simulink library "M160_lib"  (Simulink 7.8)
settings: Solver=FixedStepDiscrete  StartTime=0.0  StopTime=10.0  RelTol=1e-3
PreLoadFcn:
  | update_path
undefined symbols (not defined in the file): Afr_atCool2facLambdaReqCorr_CUR_x, Afr_atCool2facLambdaReqCorr_CUR_y, Afr_atMani2facLambdaReqCorr_CUR_x, Afr_atMani2facLambdaReqCorr_CUR_y, Afr_facLambdaReqMan, Afr_facRatioMan, Afr_facStoich, Afr_flgLambdaReqOverride, Afr_flgRatioOverride, Afr_rpmEngSpdfacRelAir2facLambdaReqBase_MAP_x, Afr_rpmEngSpdfacRelAir2facLambdaReqBase_MAP_y, Afr_rpmEngSpdfacRelAir2facLambdaReqBase_MAP_z, Ais_flgAirInjReacPumpOverride, Ais_stAirInjReacPumpMan, Amc_flgAirMassFlowOverride, Amc_uSens2AirMassFlow_CUR_x, Amc_uSens2AirMassFlow_CUR_y, Amc_uSensMaxValid, Amc_uSensMinValid, Amf_facRelAirMan, Amf_flgAirMassPerStrOverride, Amf_flgRelAirOverride, Amf_flgSwitch2AirMassFlowMeter, Amf_mAirPerStrMan, Amf_pManiEngSpd2facRelAirCorr_MAP_x, Amf_pManiEngSpd2facRelAirCorr_MAP_y, Amf_pManiEngSpd2facRelAirCorr_MAP_z, Amf_rpmEngSpd2facTempCorr_CUR_x, Amf_rpmEngSpd2facTempCorr_CUR_y, Amf_shcSpecGasConst_C, Amf_volEngDisp_C, Apv_facAirPumpRateMan, Apv_factor, Apv_flgAirPumpRateOverride, Apv_tiPeriod_C, Bvc_rVoltDivHigh, Bvc_rVoltDivLow, Bvc_uBattMax, Bvc_uBattMin, CDRV_E_OK_, Cov_facChOverVlvRateMan, Cov_factor, Cov_flgChOverVlvRateOverride, Cov_tiPeriod_C, Cpc_atManiTmp2facPresCorr_CUR_x, Cpc_atManiTmp2facPresCorr_CUR_y, Cpc_flgPChargeOverride, Cpc_uSens2pManiBase_CUR_x, Cpc_uSens2pManiBase_CUR_y, Ctc_rPullUp_C, Ctc_rSens2atCool_CUR_x, Ctc_rSens2atCool_CUR_y, Ctc_uSensMaxValid, Ctc_uSensMinValid, Ctc_uSupply, Doh_OutputDiagnosisOverride, dummy_facAirPumpRateReq, dummy_facChOverVlvRateReq, dummy_flgInterCoolerOverride, dummy_flgKl50Override ... (+243)
libraries: simulink x36, ehooks_lib x3
(part 3 of 8)

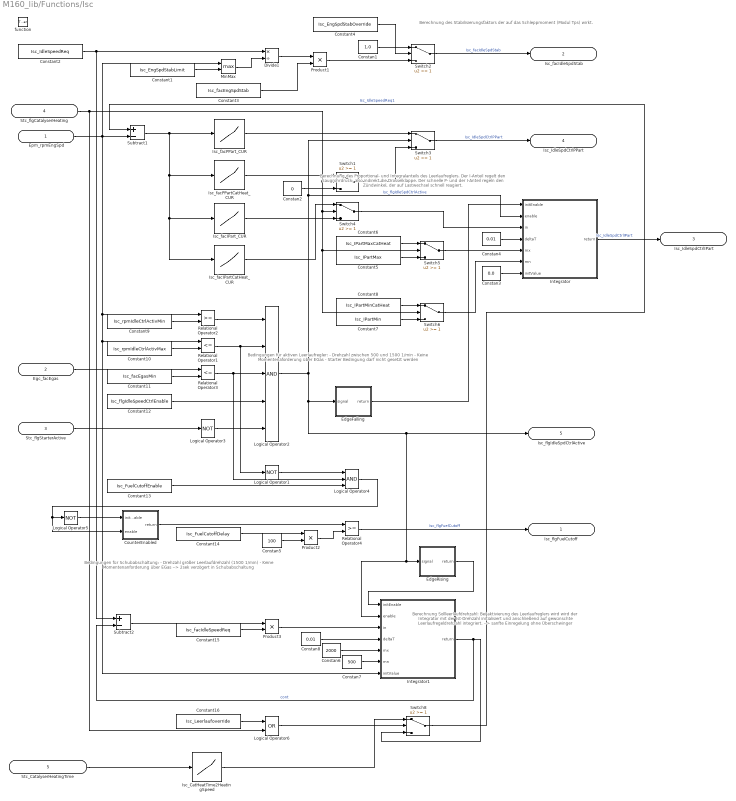
== system M160_lib/Functions/Isc ==
  note: Berechnung des Stabilisierungsfaktors der auf das Schleppmoment (Modul Tps) wirkt.
  note: Berechnung des Proportional- und Integralanteils des Leerlaufreglers.
      | Der I-Anteil regelt den Saugrohrdruck, also indirekt die Drosselklappe.
      | Der schnelle P- und der I-Anteil regeln den Zündwinkel, der auf
      | Lastwechsel schnell reagiert.
  note: Bedingungen für aktiven Leerlaufregler:
      | - Drehzahl zwischen 500 und 1500 1/min
      | - Keine Momentenaforderung über EGas
      | - Starter Bedingung darf nicht gesetzt werden
  note: Bedingungen für Schubabschaltung:
      | - Drehzahl größer Leerlaufdrehzahl (1500 1/min)
      | - Keine Momentenanforderung über EGas
      | --> 2sek verzögert in Schubabschaltung
  note: Berechnung Sollleerlaufdrehzahl:
      | Bei aktivierung des Leerlaufreglers wird
      | wird der Integrator mit der Ist-Drehzahl
      | initialisiert und anschließend auf gewünschte
      | Leerlaufregeldrehzahl integriert.
      | --> sanfte Einregelung ohne Überschwinger
  Epm_rpmEngSpd : Inport
  Egc_facEgas : Inport  Port=2
  Stc_flgStarterActive : Inport  Port=3
  Stc_flgCatalyserHeating : Inport  Port=4
  Stc_CatalyserHeatingTime : Inport  Port=5
  function : TriggerPort  TriggerType=function-call
  Constan1 : Constant  Value=1.0  OutDataTypeStr=single
  Constan2 : Constant  Value=0  OutDataTypeStr=single
  Constan3 : Constant  Value=0.0  OutDataTypeStr=single
  Constan4 : Constant  Value=0.01  OutDataTypeStr=single
  Constan5 : Constant  Value=100  OutDataTypeStr=single
  Constan6 : Constant  Value=2000  OutDataTypeStr=single
  Constan7 : Constant  Value=500  OutDataTypeStr=single
  Constan8 : Constant  Value=0.01  OutDataTypeStr=single
  Constant1 : Constant  Value=Isc_EngSpdStabLimit
  Constant10 : Constant  Value=Isc_rpmIdleCtrlActivMax
  Constant11 : Constant  Value=Isc_facEgasMin
  Constant12 : Constant  Value=Isc_flgIdleSpeedCtrlEnable
  Constant13 : Constant  Value=Isc_FuelCutoffEnable
  Constant14 : Constant  Value=Isc_FuelCutoffDelay
  Constant15 : Constant  Value=Isc_facIdleSpeedReq
  Constant16 : Constant  Value=Isc_Leerlaufoverride
  Constant2 : Constant  Value=Isc_IdleSpeedReq
  Constant3 : Constant  Value=Isc_facEngSpdStab
  Constant4 : Constant  Value=Isc_EngSpdStabOverride
  Constant5 : Constant  Value=Isc_IPartMax
  Constant6 : Constant  Value=Isc_IPartMaxCatHeat
  Constant7 : Constant  Value=Isc_IPartMin
  Constant8 : Constant  Value=Isc_IPartMinCatHeat
  Constant9 : Constant  Value=Isc_rpmIdleCtrlActivMin
  CounterEnabled : Subsystem
      mask Description: Counter
      mask Display: image(imread('CounterEnabled.jpg'))
  Divide1 : Product  Inputs=*/  OutDataTypeStr=Inherit: Same as first input
  EdgeFalling : Subsystem
      mask Description: EdgeFalling
      mask Display: image(imread('EdgeFalling.jpg'))
  EdgeRising : Subsystem
      mask Description: EdgeRising
      mask Display: image(imread('EdgeRising.jpg'))
  Integrator : Subsystem
      mask Description: Integrator
      mask Display: image(imread('Integrator.jpg'))
  Integrator1 : Subsystem
      mask Description: Integrator
      mask Display: image(imread('Integrator.jpg'))
  Isc_CatHeatTime2HeatingSpeed : Lookup_n-D  NumberOfTableDimensions=1  BreakpointsForDimension1=Isc_CatHeatTime2HeatingSpeed_x  Table=Isc_CatHeatTime2HeatingSpeed_y  ExtrapMethod=Clip  InputSameDT=on
  Isc_facIPartCatHeat_CUR : Lookup_n-D  NumberOfTableDimensions=1  BreakpointsForDimension1=Isc_facIPartCatHeat_CUR_x  Table=Isc_facIPartCatHeat_CUR_y  ExtrapMethod=Clip  InputSameDT=on
  Isc_facIPart_CUR : Lookup_n-D  NumberOfTableDimensions=1  BreakpointsForDimension1=Isc_facIPart_CUR_x  Table=Isc_facIPart_CUR_y  ExtrapMethod=Clip  InputSameDT=on
  Isc_facPPartCatHeat_CUR : Lookup_n-D  NumberOfTableDimensions=1  BreakpointsForDimension1=Isc_facPPartCatHeat_CUR_x  Table=Isc_facPPartCatHeat_CUR_y  ExtrapMethod=Clip  InputSameDT=on
  Isc_facPPart_CUR : Lookup_n-D  NumberOfTableDimensions=1  BreakpointsForDimension1=Isc_facPPart_CUR_x  Table=Isc_facPPart_CUR_y  ExtrapMethod=Clip  InputSameDT=on
  Logical Operator1 : Logic  Operator=NOT  AllPortsSameDT=off  OutDataTypeStr=boolean
  Logical Operator2 : Logic  Inputs=5  AllPortsSameDT=off  OutDataTypeStr=boolean
  Logical Operator3 : Logic  Operator=NOT  AllPortsSameDT=off  OutDataTypeStr=boolean
  Logical Operator4 : Logic  Inputs=3  AllPortsSameDT=off  OutDataTypeStr=boolean
  Logical Operator5 : Logic  Operator=NOT  AllPortsSameDT=off  OutDataTypeStr=boolean
  Logical Operator6 : Logic  Operator=OR  AllPortsSameDT=off  OutDataTypeStr=boolean
  MinMax : MinMax  Function=max  Inputs=2
  Product1 : Product  OutDataTypeStr=Inherit: Same as first input
  Product2 : Product  OutDataTypeStr=Inherit: Same as first input
  Product3 : Product  OutDataTypeStr=Inherit: Same as first input
  Relational Operator1 : RelationalOperator  Operator=<=  OutDataTypeStr=boolean
  Relational Operator2 : RelationalOperator  OutDataTypeStr=boolean
  Relational Operator3 : RelationalOperator  Operator=<=  OutDataTypeStr=boolean
  Relational Operator4 : RelationalOperator  OutDataTypeStr=boolean
  Subtract1 : Sum  Inputs=+-  OutDataTypeStr=Inherit: Same as first input
  Subtract2 : Sum  Inputs=+-  OutDataTypeStr=Inherit: Same as first input
  Switch{1..6,8} (7 alike) : Switch  Threshold=1
  Isc_flgFuelCutoff : Outport
  Isc_facIdleSpdStab : Outport  Port=2
  Isc_IdleSpdCtrlIPart : Outport  Port=3
  Isc_IdleSpdCtrlPPart : Outport  Port=4
  Isc_flgIdleSpdCtrlActive : Outport  Port=5
  wires:
  Constant2/1 -> Divide1/1, Subtract2/1
  MinMax/1 -> Divide1/2
  Constant1/1 -> MinMax/2
  Epm_rpmEngSpd/1 -> MinMax/1, Subtract1/2, Relational Operator2/1, Relational Operator1/1, Integrator1/7(initValue)
  Divide1/1 -> Product1/1
  Constant3/1 -> Product1/2
  Product1/1 -> Switch2/3
  Constan1/1 -> Switch2/1
  Constant4/1 -> Switch2/2
  Switch2/1 -> Isc_facIdleSpdStab/1  "Isc_facIdleSpdStab"
  Subtract1/1 -> Isc_facPPart_CUR/1, Isc_facPPartCatHeat_CUR/1, Isc_facIPart_CUR/1, Isc_facIPartCatHeat_CUR/1
  Constan2/1 -> Switch1/3
  Switch1/1 -> Switch3/3
  Switch3/1 -> Isc_IdleSpdCtrlPPart/1  "Isc_IdleSpdCtrlPPart"
  Stc_flgCatalyserHeating/1 -> Switch1/2, Switch4/2, Switch5/2, Switch6/2, Logical Operator6/2
  Isc_facPPartCatHeat_CUR/1 -> Switch1/1
  Isc_facPPart_CUR/1 -> Switch3/1
  Integrator/1(return) -> Isc_IdleSpdCtrlIPart/1  "Isc_IdleSpdCtrlIPart"
  Isc_facIPart_CUR/1 -> Switch4/3
  Isc_facIPartCatHeat_CUR/1 -> Switch4/1
  Switch4/1 -> Integrator/3(in)
  Constan3/1 -> Integrator/7(initValue)
  Constan4/1 -> Integrator/4(deltaT)
  Switch5/1 -> Integrator/5(mx)
  Switch6/1 -> Integrator/6(mn)
  Constant6/1 -> Switch5/1
  Constant5/1 -> Switch5/3
  Constant8/1 -> Switch6/1
  Constant7/1 -> Switch6/3
  Constant9/1 -> Relational Operator2/2
  Constant10/1 -> Relational Operator1/2
  Egc_facEgas/1 -> Relational Operator3/1
  Constant11/1 -> Relational Operator3/2
  Stc_flgStarterActive/1 -> Logical Operator3/1
  Relational Operator2/1 -> Logical Operator2/1
  Relational Operator1/1 -> Logical Operator2/2, Logical Operator1/1
  Relational Operator3/1 -> Logical Operator2/3, Logical Operator4/2
  Logical Operator3/1 -> Logical Operator2/5
  Constant12/1 -> Logical Operator2/4
  Logical Operator2/1 -> Switch3/2, Integrator/2(enable), EdgeFalling/1(signal), Isc_flgIdleSpdCtrlActive/1, EdgeRising/1(signal), Integrator1/2(enable)  "Isc_flgIdleSpdCtrlActive"
  EdgeFalling/1(return) -> Integrator/1(initEnable)
  Logical Operator1/1 -> Logical Operator4/1
  Constant13/1 -> Logical Operator4/3
  Logical Operator4/1 -> Logical Operator5/1, CounterEnabled/2(enable)
  Logical Operator5/1 -> CounterEnabled/1(initEnable)
  CounterEnabled/1(return) -> Relational Operator4/1
  Product2/1 -> Relational Operator4/2
  Constant14/1 -> Product2/1
  Constan5/1 -> Product2/2
  Relational Operator4/1 -> Isc_flgFuelCutoff/1  "Isc_flgFuelCutoff"
  Subtract2/1 -> Product3/1
  Constant15/1 -> Product3/2
  Product3/1 -> Integrator1/3(in)
  EdgeRising/1(return) -> Integrator1/1(initEnable)
  Constan8/1 -> Integrator1/4(deltaT)
  Constan6/1 -> Integrator1/5(mx)
  Constan7/1 -> Integrator1/6(mn)
  Integrator1/1(return) -> Subtract2/2, Switch8/3  "cont"
  Constant16/1 -> Logical Operator6/1
  Logical Operator6/1 -> Switch8/2
  Stc_CatalyserHeatingTime/1 -> Isc_CatHeatTime2HeatingSpeed/1
  Isc_CatHeatTime2HeatingSpeed/1 -> Switch8/1
  Switch8/1 -> Subtract1/1  "Isc_IdleSpeedReq1"

== system M160_lib/Functions/Itc ==
  note: Systemdruck:                                                                3,8bar
      | statische Menge (Steigung):                                      145g/min
      | dynamische Menge (Punkt):     4,2mg bei 2,5ms Ansteuerung
      | min. Oeffnungszeit:                              1,6ms (ab 2,0ms linear)
      | Widerstand:                                                                14,5Ohm
      | Spannung:                                                                         14V
  Epm_rpmEngSpd : Inport
  Bvc_uBatt : Inport  Port=2
  Mpc_pManiFilt : Inport  Port=3
  Isc_flgFuelCutoff : Inport  Port=4
  Fmc_mFuel : Inport  Port=5
  Iac_flgIgnCutoff : Inport  Port=6
  Stc_facFuelCorr : Inport  Port=7
  function : TriggerPort  TriggerType=function-call
  Constan8 : Constant  Value=30  OutDataTypeStr=single
  Constant1 : Constant  Value=Itc_flgInjTimeOverride
  Constant2 : Constant  Value=Itc_tiInjOffsetMan
  Constant3 : Constant  Value=Itc_tiInjMan
  Constant4 : Constant  Value=Itc_tiInjMin
  Constant5 : Constant  Value=Itc_pManiFiltMax
  Constant6 : Constant  Value=Itc_flgInjCutoffMan
  Hysteresis_Delta_RSP : Subsystem
      mask Description: Hysteresis_Delta_RSP
      mask Display: image(imread('HysteresDeltaR.jpg'))
  Itc_mFuelMass2tiInjBase_CUR : Lookup_n-D  NumberOfTableDimensions=1  BreakpointsForDimension1=Itc_mFuelMass2tiInjBase_CUR_x  Table=Itc_mFuelMass2tiInjBase_CUR_y  ExtrapMethod=Clip  InputSameDT=on
  Itc_uBatt2tiBattDelay_CUR : Lookup_n-D  NumberOfTableDimensions=1  BreakpointsForDimension1=Itc_uBatt2tiBattDelay_CUR_x  Table=Itc_uBatt2tiBattDelay_CUR_y  ExtrapMethod=Clip  InputSameDT=on
  Logical Operator2 : Logic  Operator=OR  Inputs=7  AllPortsSameDT=off  OutDataTypeStr=boolean
  Product1 : Product  OutDataTypeStr=Inherit: Same as first input
  Relational Operator : RelationalOperator  Operator=<  OutDataTypeStr=boolean
  Relational Operator1 : RelationalOperator  Operator=<  OutDataTypeStr=boolean
  Relational Operator2 : RelationalOperator  Operator=>  OutDataTypeStr=boolean
  Subtract1 : Sum  OutDataTypeStr=Inherit: Same as first input
  Switch1 : Switch  Threshold=1
  Itc_flgInjCutoff : Outport
  Itc_tiInj : Outport  Port=2
  Itc_tiBattDelay : Outport  Port=3
  Itc_tiInjOffset : Outport  Port=4
  wires:
  Constant1/1 -> Switch1/2
  Constant3/1 -> Switch1/1
  Fmc_mFuel/1 -> Itc_mFuelMass2tiInjBase_CUR/1
  Itc_mFuelMass2tiInjBase_CUR/1 -> Product1/1  "Itc_tiInjCalc"
  Stc_facFuelCorr/1 -> Product1/2
  Product1/1 -> Subtract1/1
  Constant2/1 -> Subtract1/2, Itc_tiInjOffset/1  "Itc_tiInjOffset"
  Subtract1/1 -> Switch1/3
  Constant4/1 -> Relational Operator/2
  Switch1/1 -> Relational Operator/1, Itc_tiInj/1  "Itc_tiInj"
  Relational Operator/1 -> Logical Operator2/1
  Logical Operator2/1 -> Itc_flgInjCutoff/1  "Itc_flgInjCutoff"
  Epm_rpmEngSpd/1 -> Relational Operator1/1, Hysteresis_Delta_RSP/1(in)
  Constan8/1 -> Relational Operator1/2
  Relational Operator1/1 -> Logical Operator2/2
  Hysteresis_Delta_RSP/1(return) -> Logical Operator2/3
  Mpc_pManiFilt/1 -> Relational Operator2/1
  Constant5/1 -> Relational Operator2/2
  Relational Operator2/1 -> Logical Operator2/4
  Iac_flgIgnCutoff/1 -> Logical Operator2/5
  Constant6/1 -> Logical Operator2/6
  Isc_flgFuelCutoff/1 -> Logical Operator2/7
  Bvc_uBatt/1 -> Itc_uBatt2tiBattDelay_CUR/1
  Itc_uBatt2tiBattDelay_CUR/1 -> Itc_tiBattDelay/1  "Itc_tiBattDelay"

== system M160_lib/Functions/Lcc ==
  Epm_rpmEngSpd : Inport
  Isc_flgFuelCutoff : Inport  Port=2
  Lamsoni : Inport  Port=3
  Afr_facLambdaReq : Inport  Port=4
  Stc_flgFuelCorrActive : Inport  Port=5
  Mpc_pManiFilt : Inport  Port=6
  function : TriggerPort  TriggerType=function-call
  Constan1 : Constant  Value=1.0  OutDataTypeStr=single
  Constan2 : Constant  Value=40  OutDataTypeStr=single
  Constan8 : Constant  Value=1.0  OutDataTypeStr=single
  Constant1 : Constant  Value=Lcc_flgLambdaControlActive
  Constant4 : Constant  Value=Lcc_flgSwitch2PIDController
  Divide2 : Product  Inputs=*/  OutDataTypeStr=Inherit: Same as first input
  Logical Operator1 : Logic  Inputs=3  AllPortsSameDT=off  OutDataTypeStr=boolean
  Logical Operator2 : Logic  Operator=NOT  AllPortsSameDT=off  OutDataTypeStr=boolean
  Logical Operator3 : Logic  Operator=NOT  AllPortsSameDT=off  OutDataTypeStr=boolean
  Logical Operator4 : Logic  Operator=NOT  AllPortsSameDT=off  OutDataTypeStr=boolean
  MinMax : MinMax  Function=max  Inputs=2
  PID-Controller : Subsystem
  Relational Operator2 : RelationalOperator  Operator=<  OutDataTypeStr=boolean
  Switch1 : Switch  Threshold=1
  Switch3 : Switch  Threshold=1
  Two-point-controller : Subsystem
  Lcc_facLambdaCorr : Outport
  wires:
  Isc_flgFuelCutoff/1 -> Logical Operator2/1
  Stc_flgFuelCorrActive/1 -> Logical Operator3/1
  Logical Operator2/1 -> Logical Operator1/1
  Logical Operator3/1 -> Logical Operator1/3
  Constant1/1 -> Logical Operator1/2
  Logical Operator1/1 -> Logical Operator4/1, Two-point-controller/2(in), PID-Controller/1(in)  "Lcc_flgLambdacontrolActive_1"
  Logical Operator4/1 -> Switch1/2
  Constan8/1 -> Switch1/1
  Constant4/1 -> Switch3/2, Two-point-controller/1(Lcc_flgSwitch2PIDController), PID-Controller/2(Lcc_flgSwitch2PIDController)
  Switch1/1 -> Switch3/3
  Switch3/1 -> Lcc_facLambdaCorr/1  "Lcc_facLambdaCorr"
  Lamsoni/1 -> Relational Operator2/1, PID-Controller/4(Lamsoni)
  Afr_facLambdaReq/1 -> Relational Operator2/2, PID-Controller/5(Afr_facLambdaReq)
  Epm_rpmEngSpd/1 -> MinMax/1, Two-point-controller/4(Epm_rpmEngSpd), PID-Controller/6(Epm_rpmEngSpd)
  Constan2/1 -> Divide2/1
  Constan1/1 -> MinMax/2
  MinMax/1 -> Divide2/2
  Two-point-controller/1(Lcc_facLambdaTPCCorr) -> Switch1/3
  Relational Operator2/1 -> Two-point-controller/3(in1)
  Divide2/1 -> Two-point-controller/5(dt), PID-Controller/3(dt)
  PID-Controller/1(Lcc_facLambdaPIDController) -> Switch3/1
  Mpc_pManiFilt/1 -> PID-Controller/7(Mpc_pManiFilt)

== system M160_lib/Functions/Opm ==
  Eih_flgInputError : Inport
  Doh_flgErrorDiagnosis : Inport  Port=2
  Eoh_flgOutputError : Inport  Port=3
  ErrorCheck : Subsystem
      mask Type: Functions
      mask Description: ErrorCheck
      mask Display:
      | image(imread('OperationMode.jpg'))
      | port_label('input',1,'Eih_flgInputError')
      | port_label('input',2,'Doh_flgErrorDiagnosis')
      | port_label('input',3,'Eoh_flgOutputError')
      | port_label('input',4,'Opm_flgInputErrorMem')
      | port_label('input',5,'Opm_flgOutputErrorMem')
      | port_label('output',1,'Opm_stEngControl')
      | port_label('output',2,'Erh_flgIOErrorAct')
      | port_label('output',3,'Opm_flgIOErrorMemIn')
  OpMode : Subsystem
      mask Type: Functions
      mask Description: OpMode
      mask Display:
      | image(imread('OperationMode.jpg'))
      | port_label('input',1,'Opm_stEngControl')
      | port_label('input',2,'Erh_flgIOErrorAct')
      | port_label('input',3,'Opm_flgIOErrorMemIn')
      | port_label('output',1,'Opm_idxMode')
      | port_label('output',2,'Opm_flgInputErrorMem')
      | port_label('output',3,'Opm_flgOutputErrorMem')
  Opm_ErrorCheck : Subsystem  Tag=ECU_FcnCallTrigger_Source  Description=|  LoadFcn=ehooks_fcncalltrigger_source_block('load');  InitFcn=ehooks_fcncalltrigger_source_block('init');  StartFcn=ehooks_fcncalltrigger_source_block('start');  StopFcn=ehooks_fcncalltrigger_source_block('stop');  ClipboardFcn=ehooks_fcncalltrigger_source_block('clipboard', 0); % Second argument just needed to indicate null block. See callback handler.  mask(ECU_FcnCallTrigger_Source){ProcessName=BypEasyhooks_1ms_Pre_Proc, TaskPriority=0, TaskPeriod=1}
      | [$SL_INT_DD 20060]
      | EHOOKS ECU asynchronous function-call trigger source block.
      mask prompts: ProcessName "Process name"; TaskPriority "Task priority (0..255)"; TaskPeriod "Task sample rate (ms)"
      mask help:
      | EHOOKS ECU asynchronous function-call trigger source block.
      | The EHOOKS ECU function-call trigger source block (EHOOKS trigger block) allows Simulink model code to be integrated into the execution of the ECU software.
      mask init:
      | ehooks_fcncalltrigger_source_block('mask_init');
      settings: CopyFcn=ehooks_fcncalltrigger_source_block('copy');  DeleteFcn=ehooks_fcncalltrigger_source_block('delete');  UndoDeleteFcn=ehooks_fcncalltrigger_source_block('undo_delete');  ModelCloseFcn=ehooks_fcncalltrigger_source_block('model_close');  PreSaveFcn=ehooks_fcncalltrigger_source_block('pre_save');  PostSaveFcn=ehooks_fcncalltrigger_source_block('post_save');  NameChangeFcn=ehooks_fcncalltrigger_source_block('name_change');  DestroyFcn=ehooks_fcncalltrigger_source_block('destroy', 0); % Second argument just needed to indicate null block. See callback handler.  OpenFcn=ehooks_fcncalltrigger_source_block('open');  CloseFcn=ehooks_fcncalltrigger_source_block('close');  ParentCloseFcn=ehooks_fcncalltrigger_source_block('parent_close');  MoveFcn=ehooks_fcncalltrigger_source_block('move');
      mask Display:
      | image(imread('ehooks_fcncalltrigger_source_small.bmp', 'bmp'), [ 3 1 38 30 ])
      | port_label('Output', 1, 'BypEasyhooks_1ms_Pre_Proc')
  Opm_set : Subsystem  Tag=ECU_FcnCallTrigger_Source  Description=|  LoadFcn=ehooks_fcncalltrigger_source_block('load');  InitFcn=ehooks_fcncalltrigger_source_block('init');  StartFcn=ehooks_fcncalltrigger_source_block('start');  StopFcn=ehooks_fcncalltrigger_source_block('stop');  ClipboardFcn=ehooks_fcncalltrigger_source_block('clipboard', 0); % Second argument just needed to indicate null block. See callback handler.  mask(ECU_FcnCallTrigger_Source){ProcessName=BypEasyhooks_100ms_Pre_Proc, TaskPriority=0, TaskPeriod=1}
      | [$SL_INT_DD 20060]
      | EHOOKS ECU asynchronous function-call trigger source block.
      mask prompts: ProcessName "Process name"; TaskPriority "Task priority (0..255)"; TaskPeriod "Task sample rate (ms)"
      mask help:
      | EHOOKS ECU asynchronous function-call trigger source block.
      | The EHOOKS ECU function-call trigger source block (EHOOKS trigger block) allows Simulink model code to be integrated into the execution of the ECU software.
      mask init:
      | ehooks_fcncalltrigger_source_block('mask_init');
      settings: CopyFcn=ehooks_fcncalltrigger_source_block('copy');  DeleteFcn=ehooks_fcncalltrigger_source_block('delete');  UndoDeleteFcn=ehooks_fcncalltrigger_source_block('undo_delete');  ModelCloseFcn=ehooks_fcncalltrigger_source_block('model_close');  PreSaveFcn=ehooks_fcncalltrigger_source_block('pre_save');  PostSaveFcn=ehooks_fcncalltrigger_source_block('post_save');  NameChangeFcn=ehooks_fcncalltrigger_source_block('name_change');  DestroyFcn=ehooks_fcncalltrigger_source_block('destroy', 0); % Second argument just needed to indicate null block. See callback handler.  OpenFcn=ehooks_fcncalltrigger_source_block('open');  CloseFcn=ehooks_fcncalltrigger_source_block('close');  ParentCloseFcn=ehooks_fcncalltrigger_source_block('parent_close');  MoveFcn=ehooks_fcncalltrigger_source_block('move');
      mask Display:
      | image(imread('ehooks_fcncalltrigger_source_small.bmp', 'bmp'), [ 3 1 38 30 ])
      | port_label('Output', 1, 'BypEasyhooks_100ms_Pre_Proc')
  Opm_idxMode : Outport
  wires:
  Opm_set/1(TriggerOut) -> OpMode/Trigger
  Opm_ErrorCheck/1(TriggerOut) -> ErrorCheck/Trigger
  Eih_flgInputError/1 -> ErrorCheck/1(Eih_flgInputError)
  Doh_flgErrorDiagnosis/1 -> ErrorCheck/2(Doh_flgErrorDiagnosis)
  Eoh_flgOutputError/1 -> ErrorCheck/3(Eoh_flgOutputError)
  OpMode/1(Opm_idxMode) -> Opm_idxMode/1
  ErrorCheck/1(Opm_stEngControl) -> OpMode/1(Opm_stEngControl)
  ErrorCheck/2(Erh_flgIOErrorAct) -> OpMode/2(Erh_flgIOErrorAct)
  ErrorCheck/3(Opm_flgIOErrorMemIn) -> OpMode/3(Opm_flgIOErrorMemIn)
  OpMode/2(Opm_flgInputErrorMem) -> ErrorCheck/4(Opm_flgInputErrorMem)
  OpMode/3(Opm_flgOutputErrorMem) -> ErrorCheck/5(Opm_flgOutputErrorMem)

== system M160_lib/Functions/Stc ==
  note: Bedingungen für Motorstart:
      | - Motordrehzahl unter Grenzdrehzahl
      | - Betriebsmode normal
      | - Startersignal gesetzt
  note: Motorstart bleibt so lange aktiv bis
      | eine definierte Drehzahl erreicht ist.
  note: Kat-Heizen:
      | Wird eine bestimmte Drehzahl erreicht und wurde
      | der Motor gestartet (Starter flg gesetzt),
      | wird das Kat-Heizen (flgCatalyserHeating)
      | aktiviert. Dies bleibt für eine bestimmte Zeit aktiv
      | (Zeit über Zähler ermittelt).
  note: Bei Start des Motors ist zu berücksichtigen,
      | dass eine höhere Einspritzmenge nötig ist
      | um den Wandfilmeffekt zu kompensieren
      | und damit ein Zündbares Benzin-Luft-Gemisch
      | vorhanden ist.
      | --> erhöhung der Einspritzzeit in Abhängigkeit
      |       der Zeit (Stc_facFuelCorr_CUR).
  Epm_rpmEngSpd : Inport
  dummy_Starter : Inport  Port=2
  Opm_idxMode : Inport  Port=3
  Ctc_atCool : Inport  Port=4
  function : TriggerPort  TriggerType=function-call
  Constan1 : Constant  Value=1.0  OutDataTypeStr=single
  Constan8 : Constant  Value=1.0  OutDataTypeStr=single
  Constant1 : Constant  Value=Stc_EngSpdStartOverdrive
  Constant2 : Constant  Value=Stc_EngSpdSetCatalyserHeating
  Constant3 : Constant  Value=100  OutDataTypeStr=single
  Constant4 : Constant  Value=Stc_rpmEngSpedMax
  Constant5 : Constant  Value=Normal
  Constant6 : Constant  Value=Stc_CatalyserHeatingDelay
  Constant7 : Constant  Value=100  OutDataTypeStr=single
  CounterEnabled : Subsystem
      mask Description: Counter
      mask Display: image(imread('CounterEnabled.jpg'))
  CounterEnabled1 : Subsystem
      mask Description: Counter
      mask Display: image(imread('CounterEnabled.jpg'))
  Divide1 : Product  Inputs=*/  OutDataTypeStr=Inherit: Same as first input
  Divide2 : Product  Inputs=*/  OutDataTypeStr=Inherit: Same as first input
  Logical Operator1 : Logic  Inputs=3  AllPortsSameDT=off  OutDataTypeStr=boolean
  Logical Operator2 : Logic  AllPortsSameDT=off  OutDataTypeStr=boolean
  Logical Operator3 : Logic  Operator=NOT  AllPortsSameDT=off  OutDataTypeStr=boolean
  Logical Operator4 : Logic  AllPortsSameDT=off  OutDataTypeStr=boolean
  Logical Operator5 : Logic  AllPortsSameDT=off  OutDataTypeStr=boolean
  Logical Operator6 : Logic  Operator=NOT  AllPortsSameDT=off  OutDataTypeStr=boolean
  RSFlipFlop : Subsystem
      mask Description: RSFlipFlop
      mask Display: image(imread('RSFlipFlop.jpg'))
  RSFlipFlop1 : Subsystem
      mask Description: RSFlipFlop
      mask Display: image(imread('RSFlipFlop.jpg'))
  RSFlipFlop2 : Subsystem
      mask Description: RSFlipFlop
      mask Display: image(imread('RSFlipFlop.jpg'))
  RSFlipFlop3 : Subsystem
      mask Description: RSFlipFlop
      mask Display: image(imread('RSFlipFlop.jpg'))
  Relational Operator1 : RelationalOperator  Operator===  OutDataTypeStr=boolean
  Relational Operator2 : RelationalOperator  Operator=<  OutDataTypeStr=boolean
  Relational Operator3 : RelationalOperator  Operator=<  OutDataTypeStr=boolean
  Relational Operator4 : RelationalOperator  OutDataTypeStr=boolean
  Relational Operator5 : RelationalOperator  OutDataTypeStr=boolean
  Relational Operator6 : RelationalOperator  Operator=~=  OutDataTypeStr=boolean
  Stc_facFuelCorr_MAP : Lookup_n-D  BreakpointsForDimension1=Stc_facFuelCorr_MAP_x  BreakpointsForDimension2=Stc_facFuelCorr_MAP_y  Table=Stc_facFuelCorr_MAP_z  ExtrapMethod=Clip  InputSameDT=on
  Switch3 : Switch  Threshold=1
  Terminator{,1..3} (4 alike) : Terminator
  Stc_flgFuelCorrActive : Outport
  Stc_flgStarterActive : Outport  Port=2
  Stc_CatalyserHeatingTime : Outport  Port=3
  Stc_facFuelCorr : Outport  Port=4
  Stc_stStarter : Outport  Port=5
  Stc_flgCatalyserHeating : Outport  Port=6
  wires:
  RSFlipFlop/2(nq) -> Terminator/1
  Epm_rpmEngSpd/1 -> Relational Operator2/1, Relational Operator3/1, Relational Operator4/1
  Relational Operator2/1 -> Logical Operator1/1
  Constant4/1 -> Relational Operator2/2
  dummy_Starter/1 -> Logical Operator1/2
  Opm_idxMode/1 -> Relational Operator1/1
  Constant5/1 -> Relational Operator1/2
  Relational Operator1/1 -> Logical Operator1/3
  Logical Operator1/1 -> Stc_stStarter/1, RSFlipFlop/1(s)  "Stc_stStarter"
  Constant1/1 -> Relational Operator3/2
  RSFlipFlop/1(q) -> Logical Operator2/1
  Relational Operator3/1 -> Logical Operator2/2, Logical Operator3/1
  Logical Operator3/1 -> RSFlipFlop/2(r)
  Logical Operator2/1 -> Stc_flgStarterActive/1, RSFlipFlop1/1(s), RSFlipFlop3/1(s)  "Stc_flgStarterActive"
  RSFlipFlop1/2(nq) -> Terminator1/1
  Constant2/1 -> Relational Operator4/2
  Relational Operator4/1 -> Logical Operator4/2
  RSFlipFlop1/1(q) -> Logical Operator4/1  "Stc_StarterHold"
  RSFlipFlop2/2(nq) -> Terminator2/1
  Logical Operator4/1 -> RSFlipFlop2/1(s)
  RSFlipFlop2/1(q) -> Stc_flgCatalyserHeating/1, Logical Operator5/1  "Stc_flgCatalyserHeating"
  CounterEnabled/1(return) -> Divide2/1
  Constant3/1 -> Divide2/2
  Divide2/1 -> Relational Operator5/1, Stc_CatalyserHeatingTime/1  "Stc_CatalyserHeatingTime"
  Constant6/1 -> Relational Operator5/2
  Relational Operator5/1 -> RSFlipFlop1/2(r), RSFlipFlop2/2(r), Logical Operator6/1, CounterEnabled/1(initEnable), RSFlipFlop3/2(r), CounterEnabled1/1(initEnable)  "Stc_Memory"
  Logical Operator6/1 -> Logical Operator5/2
  Logical Operator5/1 -> CounterEnabled/2(enable)
  RSFlipFlop3/2(nq) -> Terminator3/1
  CounterEnabled1/1(return) -> Divide1/1
  Constant7/1 -> Divide1/2
  RSFlipFlop3/1(q) -> CounterEnabled1/2(enable), Switch3/2
  Divide1/1 -> Stc_facFuelCorr_MAP/1
  Ctc_atCool/1 -> Stc_facFuelCorr_MAP/2
  Constan8/1 -> Switch3/3
  Stc_facFuelCorr_MAP/1 -> Switch3/1
  Switch3/1 -> Stc_facFuelCorr/1, Relational Operator6/1  "Stc_facFuelCorr"
  Relational Operator6/1 -> Stc_flgFuelCorrActive/1  "Stc_flgFuelCorrActive"
  Constan1/1 -> Relational Operator6/2

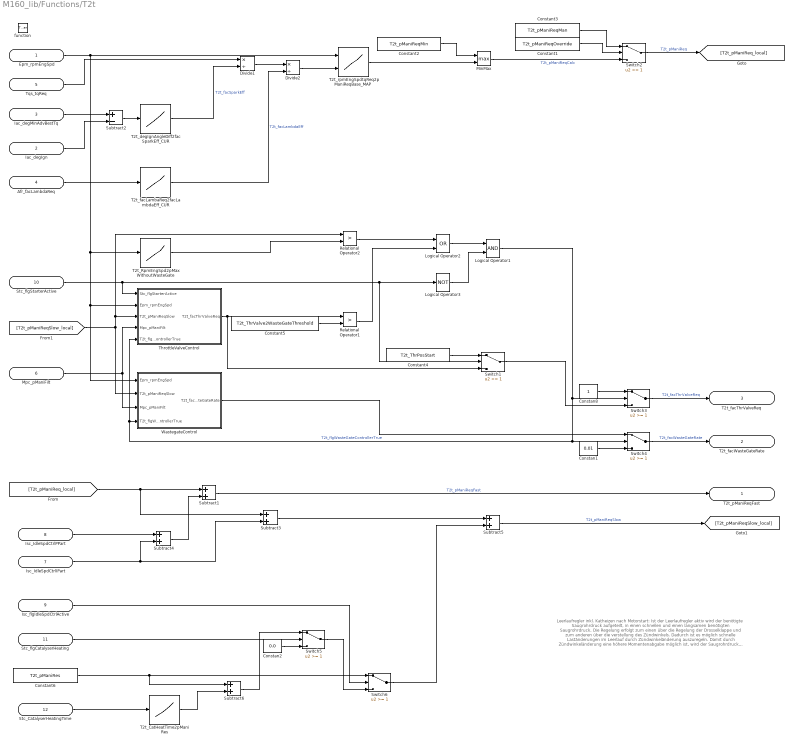
== system M160_lib/Functions/T2t ==
  note: Leerlaufregler inkl. Katheizen nach Motorstart:
      | Ist der Leerlaufregler aktiv wird der benötigte
      | Saugrohrdruck aufgeteilt, in einen schnellen
      | und einen langsamen benötigten Saugrohrdruck.
      | Die Regelung erfolgt zum einen über die
      | Regelung der Drosselklappe und zum anderen
      | über die verstellung des Zündwinkels.
      | Dadurch ist es möglich schnelle
      | Laständerungen im Leerlauf
      | durch Zündwinkeländerung auszuregeln.
      | Damit durch Zündwinkeländerung eine höhere
      | Momentenabgabe möglich ist, wird der
      | Saugrohrdruck erhöht um eine spätere
      | Zündung zu erhalten. Der
      | Zündwinkelwirkungsgrad wird niedriger.
      | Dadurch ist eine Momentenreserve vorhanden.
      |
      |
      | Der langsame Saugrohrdruck wird durch den
      | I-Anteil des Leerlaufreglers korrigiert.
      | Außerdem wird die Saugrohrdruckreserve addiert.
      | Der schnelle Saugrohrdruck wird durch den
      | P- und den I-Anteil des Leerlaufreglers korrigiert.
  Epm_rpmEngSpd : Inport
  Iac_degIgn : Inport  Port=2
  Iac_degMinAdvBestTq : Inport  Port=3
  Afr_facLambdaReq : Inport  Port=4
  Tqs_tqReq : Inport  Port=5
  Mpc_pManiFilt : Inport  Port=6
  Isc_IdleSpdCtrlIPart : Inport  Port=7
  Isc_IdleSpdCtrlPPart : Inport  Port=8
  Isc_flgIdleSpdCtrlActive : Inport  Port=9
  Stc_flgStarterActive : Inport  Port=10
  Stc_flgCatalyserHeating : Inport  Port=11
  Stc_CatalyserHeatingTime : Inport  Port=12
  function : TriggerPort  TriggerType=function-call
  Constan1 : Constant  Value=0.01  OutDataTypeStr=single
  Constan2 : Constant  Value=0.0  OutDataTypeStr=single
  Constan8 : Constant  OutDataTypeStr=single
  Constant1 : Constant  Value=T2t_pManiReqOverride
  Constant2 : Constant  Value=T2t_pManiReqMin
  Constant3 : Constant  Value=T2t_pManiReqMan
  Constant4 : Constant  Value=T2t_ThrPosStart
  Constant5 : Constant  Value=T2t_ThrValve2WasteGateThreshold
  Constant6 : Constant  Value=T2t_pManiRes
  Divide1 : Product  Inputs=*/  OutDataTypeStr=Inherit: Same as first input
  Divide2 : Product  Inputs=*/  OutDataTypeStr=Inherit: Same as first input
  Logical Operator1 : Logic  AllPortsSameDT=off  OutDataTypeStr=boolean
  Logical Operator2 : Logic  Operator=OR  AllPortsSameDT=off  OutDataTypeStr=boolean
  Logical Operator3 : Logic  Operator=NOT  AllPortsSameDT=off  OutDataTypeStr=boolean
  MinMax : MinMax  Function=max  Inputs=2
  Relational Operator1 : RelationalOperator  Operator=>  OutDataTypeStr=boolean
  Relational Operator2 : RelationalOperator  Operator=>  OutDataTypeStr=boolean
  Subtract{1,3..6} (5 alike) : Sum  OutDataTypeStr=Inherit: Same as first input
  Subtract2 : Sum  Inputs=+-  OutDataTypeStr=Inherit: Same as first input
  Switch{1..6} (6 alike) : Switch  Threshold=1
  T2t_CatHeatTime2pManiRes : Lookup_n-D  NumberOfTableDimensions=1  BreakpointsForDimension1=T2t_CatHeatTime2pManiRes_x  Table=T2t_CatHeatTime2pManiRes_y  ExtrapMethod=Clip  InputSameDT=on
  T2t_RpmEngSpd2pMaxWithoutWasteGate : Lookup_n-D  NumberOfTableDimensions=1  BreakpointsForDimension1=T2t_RpmEngSpd2pMaxWithoutWasteGate_x  Table=T2t_RpmEngSpd2pMaxWithoutWasteGate_y  ExtrapMethod=Clip  InputSameDT=on
  T2t_degIgnAngleDiff2facSparkEff_CUR : Lookup_n-D  NumberOfTableDimensions=1  BreakpointsForDimension1=T2t_degIgnAngleDiff2facSparkEff_CUR_x  Table=T2t_degIgnAngleDiff2facSparkEff_CUR_y  ExtrapMethod=Clip  InputSameDT=on
  T2t_facLambaReq2facLambdaEff_CUR : Lookup_n-D  NumberOfTableDimensions=1  BreakpointsForDimension1=T2t_facLambaReq2facLambdaEff_CUR_x  Table=T2t_facLambaReq2facLambdaEff_CUR_y  ExtrapMethod=Clip  InputSameDT=on
  T2t_rpmEngSpdtqReq2pManiReqBase_MAP : Lookup_n-D  BreakpointsForDimension1=T2t_rpmEngSpdtqReq2pManiReqBase_MAP_x  BreakpointsForDimension2=T2t_rpmEngSpdtqReq2pManiReqBase_MAP_y  Table=T2t_rpmEngSpdtqReq2pManiReqBase_MAP_z  ExtrapMethod=Clip  InputSameDT=on
  ThrottleValveControl : Subsystem
  WastegateControl : Subsystem
  T2t_pManiReqFast : Outport
  T2t_facWasteGateRate : Outport  Port=2
  T2t_facThrValveReq : Outport  Port=3
  wires:
  Constant1/1 -> Switch2/2
  Constant3/1 -> Switch2/1
  MinMax/1 -> Switch2/3  "T2t_pManiReqCalc"
  Constant2/1 -> MinMax/1
  T2t_rpmEngSpdtqReq2pManiReqBase_MAP/1 -> MinMax/2
  Switch2/1 -> [T2t_pManiReq_local]  "T2t_pManiReq"
  Divide2/1 -> T2t_rpmEngSpdtqReq2pManiReqBase_MAP/2
  Divide1/1 -> Divide2/1
  Epm_rpmEngSpd/1 -> T2t_rpmEngSpdtqReq2pManiReqBase_MAP/1, T2t_RpmEngSpd2pMaxWithoutWasteGate/1, ThrottleValveControl/2(Epm_rpmEngSpd), WastegateControl/1(Epm_rpmEngSpd)
  Tqs_tqReq/1 -> Divide1/1
  Iac_degMinAdvBestTq/1 -> Subtract2/1
  Iac_degIgn/1 -> Subtract2/2
  Subtract2/1 -> T2t_degIgnAngleDiff2facSparkEff_CUR/1
  T2t_degIgnAngleDiff2facSparkEff_CUR/1 -> Divide1/2  "T2t_facSparkEff"
  Afr_facLambdaReq/1 -> T2t_facLambaReq2facLambdaEff_CUR/1
  T2t_facLambaReq2facLambdaEff_CUR/1 -> Divide2/2  "T2t_facLambdaEff"
  T2t_RpmEngSpd2pMaxWithoutWasteGate/1 -> Relational Operator2/2
  Relational Operator2/1 -> Logical Operator2/1
  Stc_flgStarterActive/1 -> Logical Operator3/1, Switch1/2, ThrottleValveControl/1(Stc_flgStarterActive)
  Logical Operator2/1 -> Logical Operator1/1
  Logical Operator3/1 -> Logical Operator1/2
  Constant4/1 -> Switch1/1
  Logical Operator1/1 -> Switch3/2, Switch4/2, ThrottleValveControl/5(T2t_flgWasteGateControllerTrue), WastegateControl/4(T2t_flgWasteGateControllerTrue)  "T2t_flgWasteGateControllerTrue"
  Constan8/1 -> Switch3/1
  Switch1/1 -> Switch3/3
  Switch3/1 -> T2t_facThrValveReq/1  "T2t_facThrValveReq"
  Relational Operator1/1 -> Logical Operator2/2
  Constant5/1 -> Relational Operator1/2
  Switch4/1 -> T2t_facWasteGateRate/1  "T2t_facWasteGateRate"
  Constan1/1 -> Switch4/3
  [T2t_pManiReq_local] -> Subtract1/1, Subtract3/1
  Subtract4/1 -> Subtract1/2
  Isc_IdleSpdCtrlPPart/1 -> Subtract4/1
  Isc_IdleSpdCtrlIPart/1 -> Subtract4/2, Subtract3/2
  Subtract1/1 -> T2t_pManiReqFast/1  "T2t_pManiReqFast"
  [T2t_pManiReqSlow_local] -> Relational Operator2/1, ThrottleValveControl/3(T2t_pManiReqSlow), WastegateControl/2(T2t_pManiReqSlow)
  Subtract3/1 -> Subtract5/1
  Subtract5/1 -> [T2t_pManiReqSlow_local]  "T2t_pManiReqSlow"
  Stc_CatalyserHeatingTime/1 -> T2t_CatHeatTime2pManiRes/1
  Constant6/1 -> Subtract6/1, Switch6/1
  T2t_CatHeatTime2pManiRes/1 -> Subtract6/2
  Constan2/1 -> Switch5/3
  Stc_flgCatalyserHeating/1 -> Switch5/2
  Subtract6/1 -> Switch5/1
  Switch5/1 -> Switch6/3
  Isc_flgIdleSpdCtrlActive/1 -> Switch6/2
  Switch6/1 -> Subtract5/2
  ThrottleValveControl/1(T2t_facThrValveReq) -> Relational Operator1/1, Switch1/3
  Mpc_pManiFilt/1 -> ThrottleValveControl/4(Mpc_pManiFilt), WastegateControl/3(Mpc_pManiFilt)
  WastegateControl/1(T2t_facWasteGateRate) -> Switch4/1

== system M160_lib/Functions/Tqs ==
  Epm_rpmEngSpd : Inport
  Amf_facRelAir : Inport  Port=2
  Ctc_atCool : Inport  Port=3
  Egc_facEgas : Inport  Port=4
  Isc_facIdleSpdStab : Inport  Port=5
  function : TriggerPort  TriggerType=function-call
  Constant1 : Constant  Value=Tqs_flgTorqueReqOverride
  Constant3 : Constant  Value=Tqs_tqReqMan
  EngSpdControl : Subsystem
  Product1 : Product  OutDataTypeStr=Inherit: Same as first input
  Product2 : Product  OutDataTypeStr=Inherit: Same as first input
  Subtract : Sum  OutDataTypeStr=Inherit: Same as first input
  Subtract1 : Sum  OutDataTypeStr=Inherit: Same as first input
  Subtract2 : Sum  Inputs=+-  OutDataTypeStr=Inherit: Same as first input
  Subtract3 : Sum  OutDataTypeStr=Inherit: Same as first input
  Switch1 : Switch  Threshold=1
  Tqs_atCool2tqDrag_CUR : Lookup_n-D  NumberOfTableDimensions=1  BreakpointsForDimension1=Tqs_atCool2tqDrag_CUR_x  Table=Tqs_atCool2tqDrag_CUR_y  ExtrapMethod=Clip  InputSameDT=on
  Tqs_rpmEngSpd2tqMax_CUR : Lookup_n-D  NumberOfTableDimensions=1  BreakpointsForDimension1=Tqs_rpmEngSpd2tqMax_CUR_x  Table=Tqs_rpmEngSpd2tqMax_CUR_y  ExtrapMethod=Clip  InputSameDT=on
  Tqs_rpmEngSpdfacEgas2facEgasFilt_MAP : Lookup_n-D  BreakpointsForDimension1=Tqs_rpmEngSpdfacEgas2facEgasFilt_MAP_x  BreakpointsForDimension2=Tqs_rpmEngSpdfacEgas2facEgasFilt_MAP_y  Table=Tqs_rpmEngSpdfacEgas2facEgasFilt_MAP_z  ExtrapMethod=Clip  InputSameDT=on
  Tqs_rpmEngSpdfacRelAir2tqDrag_MAP : Lookup_n-D  BreakpointsForDimension1=Tqs_rpmEngSpdfacRelAir2tqDrag_MAP_x  BreakpointsForDimension2=Tqs_rpmEngSpdfacRelAir2tqDrag_MAP_y  Table=Tqs_rpmEngSpdfacRelAir2tqDrag_MAP_z  ExtrapMethod=Clip  InputSameDT=on
  Tqs_tqMin : Terminator
  Tqs_tqReq : Outport
  wires:
  Constant3/1 -> Switch1/1
  Constant1/1 -> Switch1/2
  Epm_rpmEngSpd/1 -> EngSpdControl/1(Epm_rpmEngSpd), Tqs_rpmEngSpdfacEgas2facEgasFilt_MAP/1, Tqs_rpmEngSpd2tqMax_CUR/1, Tqs_rpmEngSpdfacRelAir2tqDrag_MAP/1
  Egc_facEgas/1 -> EngSpdControl/2(Egc_facEgas), Tqs_rpmEngSpdfacEgas2facEgasFilt_MAP/2
  Amf_facRelAir/1 -> Tqs_rpmEngSpdfacRelAir2tqDrag_MAP/2
  Ctc_atCool/1 -> Tqs_atCool2tqDrag_CUR/1
  Tqs_rpmEngSpdfacRelAir2tqDrag_MAP/1 -> Subtract/1
  Tqs_atCool2tqDrag_CUR/1 -> Subtract/2
  Switch1/1 -> Tqs_tqReq/1  "Tqs_tqReq"
  Tqs_rpmEngSpdfacEgas2facEgasFilt_MAP/1 -> Product1/1  "Tqs_facEgasFilt"
  Subtract2/1 -> Product1/2
  Tqs_rpmEngSpd2tqMax_CUR/1 -> Subtract2/1  "Tqs_tqMax"
  Product1/1 -> Subtract1/1
  Product2/1 -> Subtract2/2, Subtract1/2, Tqs_tqMin/1  "Tqs_tqMin"
  Subtract/1 -> Product2/1  "Tqs_tqDrag"
  Isc_facIdleSpdStab/1 -> Product2/2
  EngSpdControl/1(Tqs_tqIdleSpdCtrlCorr) -> Subtract3/1
  Subtract1/1 -> Subtract3/2
  Subtract3/1 -> Switch1/3  "Tqs_tqReqCalc"

== system M160_lib/Sensors/Amc ==
  function : TriggerPort  TriggerType=function-call
  Amc_uSens2AirMassFlow_CUR : Lookup_n-D  NumberOfTableDimensions=1  BreakpointsForDimension1=Amc_uSens2AirMassFlow_CUR_x  BreakpointsForDimension1DataTypeStr=Inherit: Inherit from 'Breakpoint data'  Table=Amc_uSens2AirMassFlow_CUR_y  TableDataTypeStr=Inherit: Inherit from 'Table data'  ExtrapMethod=Clip  OutDataTypeStr=Inherit: Inherit from 'Table data'  InputSameDT=on
  Constant1 : Constant  Value=0  OutDataTypeStr=boolean
  Constant4 : Constant  Value=Amc_flgAirMassFlowOverride
  G1_ADC_Input_Receive : Subsystem  LoadFcn=ehooks_medc17flex_devlib_io_block('load');  InitFcn=ehooks_medc17flex_devlib_io_block('init');  StartFcn=ehooks_medc17flex_devlib_io_block('start');  StopFcn=ehooks_medc17flex_devlib_io_block('stop');  ClipboardFcn=ehooks_medc17flex_devlib_io_block('clipboard', 0); % Second argument just needed to indicate null block. See callback handler.  mask{ChannelName=I_A_AN21}
      mask prompts: ChannelName "Channel name"
      mask init:
      | ehooks_medc17flex_devlib_io_block('mask_init');
      settings: AttributesFormatString=Channel name: '%<ChannelName>'  CopyFcn=ehooks_medc17flex_devlib_io_block('copy');  DeleteFcn=ehooks_medc17flex_devlib_io_block('delete');  UndoDeleteFcn=ehooks_medc17flex_devlib_io_block('undo_delete');  ModelCloseFcn=ehooks_medc17flex_devlib_io_block('model_close');  PreSaveFcn=ehooks_medc17flex_devlib_io_block('pre_save');  PostSaveFcn=ehooks_medc17flex_devlib_io_block('post_save');  NameChangeFcn=ehooks_medc17flex_devlib_io_block('name_change');  DestroyFcn=ehooks_medc17flex_devlib_io_block('destroy', 0); % Second argument just needed to indicate null block. See callback handler.  OpenFcn=ehooks_medc17flex_devlib_io_block('open');  CloseFcn=ehooks_medc17flex_devlib_io_block('close');  ParentCloseFcn=ehooks_medc17flex_devlib_io_block('parent_close');  MoveFcn=ehooks_medc17flex_devlib_io_block('move');
      mask StyleString: popup(<empty>|I_A_AN01|I_A_AN02|I_A_AN03|I_A_AN05|I_A_AN06|I_A_AN07|I_A_AN08|I_A_AN10|I_A_AN11|I_A_AN12|I_A_AN13|I_A_AN14|I_A_AN15|I_A_AN16|I_A_AN17|I_A_AN18|I_A_AN19|I_A_AN20|I_A_AN21|I_A_AN23|I_A_AN32|I_A_AN35|I_A_AN36|I_A_AN37|I_A_AN39|I_A_AN100|I_A_AN101|I_A_AN103|I_A_AN104|I_A_AN105|I_A_AN106)
      mask Display: image(imread('Input_Analog.jpg'))
  Interval Test : simulink/Logic and Bit Operations/Interval Test  IntervalClosedRight=on  uplimit=Amc_uSensMaxValid  IntervalClosedLeft=on  lowlimit=Amc_uSensMinValid  OutDataTypeStr=boolean
  Logical Operator : Logic  Operator=NOT  AllPortsSameDT=off  OutDataTypeStr=boolean
  Logical Operator1 : Logic  Operator=NOT  AllPortsSameDT=off  OutDataTypeStr=boolean
  Logical Operator3 : Logic  Operator=OR  AllPortsSameDT=off  OutDataTypeStr=boolean
  Switch2 : Switch  Threshold=1
  Amc_flgError : Outport
  Amc_AirMassFlow : Outport  Port=2
  wires:
  G1_ADC_Input_Receive/1(status) -> Logical Operator/1  "Amc_stIOError"
  G1_ADC_Input_Receive/2(uRaw) -> Amc_uSens2AirMassFlow_CUR/1, Interval Test/1  "Amc_uSens"
  Interval Test/1 -> Logical Operator1/1
  Logical Operator/1 -> Logical Operator3/1
  Logical Operator1/1 -> Logical Operator3/2
  Switch2/1 -> Amc_flgError/1  "Amc_flgError"
  Amc_uSens2AirMassFlow_CUR/1 -> Amc_AirMassFlow/1  "Amc_AirMassFlow"
  Constant1/1 -> Switch2/1
  Logical Operator3/1 -> Switch2/3
  Constant4/1 -> Switch2/2

== system M160_lib/Sensors/Bvc ==
  function : TriggerPort  TriggerType=function-call
  Constant : Constant  Value=Bvc_rVoltDivHigh
  Constant3 : Constant  Value=Bvc_rVoltDivLow
  Divide : Product  Inputs=*/  OutDataTypeStr=Inherit: Same as first input
  G1_ADC_Input_Receive : Subsystem  LoadFcn=ehooks_medc17flex_devlib_io_block('load');  InitFcn=ehooks_medc17flex_devlib_io_block('init');  StartFcn=ehooks_medc17flex_devlib_io_block('start');  StopFcn=ehooks_medc17flex_devlib_io_block('stop');  ClipboardFcn=ehooks_medc17flex_devlib_io_block('clipboard', 0); % Second argument just needed to indicate null block. See callback handler.  mask{ChannelName=I_A_AN16}
      mask prompts: ChannelName "Channel name"
      mask init:
      | ehooks_medc17flex_devlib_io_block('mask_init');
      settings: AttributesFormatString=Channel name: '%<ChannelName>'  CopyFcn=ehooks_medc17flex_devlib_io_block('copy');  DeleteFcn=ehooks_medc17flex_devlib_io_block('delete');  UndoDeleteFcn=ehooks_medc17flex_devlib_io_block('undo_delete');  ModelCloseFcn=ehooks_medc17flex_devlib_io_block('model_close');  PreSaveFcn=ehooks_medc17flex_devlib_io_block('pre_save');  PostSaveFcn=ehooks_medc17flex_devlib_io_block('post_save');  NameChangeFcn=ehooks_medc17flex_devlib_io_block('name_change');  DestroyFcn=ehooks_medc17flex_devlib_io_block('destroy', 0); % Second argument just needed to indicate null block. See callback handler.  OpenFcn=ehooks_medc17flex_devlib_io_block('open');  CloseFcn=ehooks_medc17flex_devlib_io_block('close');  ParentCloseFcn=ehooks_medc17flex_devlib_io_block('parent_close');  MoveFcn=ehooks_medc17flex_devlib_io_block('move');
      mask StyleString: popup(<empty>|I_A_AN01|I_A_AN02|I_A_AN03|I_A_AN05|I_A_AN06|I_A_AN07|I_A_AN08|I_A_AN10|I_A_AN11|I_A_AN12|I_A_AN13|I_A_AN14|I_A_AN15|I_A_AN16|I_A_AN17|I_A_AN18|I_A_AN19|I_A_AN20|I_A_AN21|I_A_AN23|I_A_AN32|I_A_AN35|I_A_AN36|I_A_AN37|I_A_AN39|I_A_AN100|I_A_AN101|I_A_AN103|I_A_AN104|I_A_AN105|I_A_AN106)
      mask Display: image(imread('Input_Analog.jpg'))
  Gain : Gain
  Interval Test : simulink/Logic and Bit Operations/Interval Test  IntervalClosedRight=on  uplimit=Bvc_uBattMax  IntervalClosedLeft=on  lowlimit=Bvc_uBattMin  OutDataTypeStr=boolean
  Logical Operator : Logic  Operator=NOT  AllPortsSameDT=off  OutDataTypeStr=boolean
  Logical Operator1 : Logic  Operator=NOT  AllPortsSameDT=off  OutDataTypeStr=boolean
  Logical Operator4 : Logic  Operator=OR  AllPortsSameDT=off  OutDataTypeStr=boolean
  Product : Product  OutDataTypeStr=Inherit: Same as first input
  Subtract : Sum  OutDataTypeStr=Inherit: Same as first input
  Bvc_flgError : Outport
  Bvc_uBatt : Outport  Port=2
  wires:
  G1_ADC_Input_Receive/1(status) -> Logical Operator/1  "Bvc_stIA"
  Interval Test/1 -> Logical Operator1/1
  Logical Operator/1 -> Logical Operator4/1
  Logical Operator1/1 -> Logical Operator4/2
  Logical Operator4/1 -> Bvc_flgError/1  "Bvc_flgError"
  Constant/1 -> Subtract/1
  Constant3/1 -> Subtract/2, Divide/2
  Subtract/1 -> Divide/1
  Product/1 -> Gain/1, Interval Test/1  "Bvc_uBattCalc"
  G1_ADC_Input_Receive/2(uRaw) -> Product/1  "Bvc_uSens"
  Divide/1 -> Product/2
  Gain/1 -> Bvc_uBatt/1  "Bvc_uBatt"

== system M160_lib/Sensors/Cpc ==
  In1 : Inport
  Mtc_atMani : Inport  Port=2
  Cpc_calc : Subsystem
      mask Type: Sensors
      mask Description: ChargingPressureCalc
      mask Display:
      | image(imread('ManifoldPressure.jpg'))
      | port_label('input',1,'Epm_rpmEngSpd')
      | port_label('input',2,'Cpc_pMani')
      | port_label('input',3,'Cpc_flgError')
      | port_label('output',1,'Cpc_pChargeFilt')
  Cpc_get : Subsystem
      mask Type: Sensors
      mask Description: ChargingPressureGet
      mask Display:
      | image(imread('ManifoldPressure.jpg'))
      | port_label('input',1,'Mtc_atMani')
      | port_label('output',1,'Cpc_flgError')
      | port_label('output',2,'Cpc_pMani')
  Cpc_pCharge_calc : Subsystem  Tag=ECU_FcnCallTrigger_Source  Description=|  LoadFcn=ehooks_fcncalltrigger_source_block('load');  InitFcn=ehooks_fcncalltrigger_source_block('init');  StartFcn=ehooks_fcncalltrigger_source_block('start');  StopFcn=ehooks_fcncalltrigger_source_block('stop');  ClipboardFcn=ehooks_fcncalltrigger_source_block('clipboard', 0); % Second argument just needed to indicate null block. See callback handler.  mask(ECU_FcnCallTrigger_Source){ProcessName=BypEasyhooks_S0_Pre_Proc, TaskPriority=0, TaskPeriod=1}
      | [$SL_INT_DD 20060]
      | EHOOKS ECU asynchronous function-call trigger source block.
      mask prompts: ProcessName "Process name"; TaskPriority "Task priority (0..255)"; TaskPeriod "Task sample rate (ms)"
      mask help:
      | EHOOKS ECU asynchronous function-call trigger source block.
      | The EHOOKS ECU function-call trigger source block (EHOOKS trigger block) allows Simulink model code to be integrated into the execution of the ECU software.
      mask init:
      | ehooks_fcncalltrigger_source_block('mask_init');
      settings: CopyFcn=ehooks_fcncalltrigger_source_block('copy');  DeleteFcn=ehooks_fcncalltrigger_source_block('delete');  UndoDeleteFcn=ehooks_fcncalltrigger_source_block('undo_delete');  ModelCloseFcn=ehooks_fcncalltrigger_source_block('model_close');  PreSaveFcn=ehooks_fcncalltrigger_source_block('pre_save');  PostSaveFcn=ehooks_fcncalltrigger_source_block('post_save');  NameChangeFcn=ehooks_fcncalltrigger_source_block('name_change');  DestroyFcn=ehooks_fcncalltrigger_source_block('destroy', 0); % Second argument just needed to indicate null block. See callback handler.  OpenFcn=ehooks_fcncalltrigger_source_block('open');  CloseFcn=ehooks_fcncalltrigger_source_block('close');  ParentCloseFcn=ehooks_fcncalltrigger_source_block('parent_close');  MoveFcn=ehooks_fcncalltrigger_source_block('move');
      mask Display:
      | image(imread('ehooks_fcncalltrigger_source_small.bmp', 'bmp'), [ 3 1 38 30 ])
      | port_label('Output', 1, 'BypEasyhooks_S0_Pre_Proc')
  Cpc_pCharge_get : Subsystem  Tag=ECU_FcnCallTrigger_Source  Description=|  LoadFcn=ehooks_fcncalltrigger_source_block('load');  InitFcn=ehooks_fcncalltrigger_source_block('init');  StartFcn=ehooks_fcncalltrigger_source_block('start');  StopFcn=ehooks_fcncalltrigger_source_block('stop');  ClipboardFcn=ehooks_fcncalltrigger_source_block('clipboard', 0); % Second argument just needed to indicate null block. See callback handler.  mask(ECU_FcnCallTrigger_Source){ProcessName=BypEasyhooks_1ms_Pre_Proc, TaskPriority=0, TaskPeriod=1}
      | [$SL_INT_DD 20060]
      | EHOOKS ECU asynchronous function-call trigger source block.
      mask prompts: ProcessName "Process name"; TaskPriority "Task priority (0..255)"; TaskPeriod "Task sample rate (ms)"
      mask help:
      | EHOOKS ECU asynchronous function-call trigger source block.
      | The EHOOKS ECU function-call trigger source block (EHOOKS trigger block) allows Simulink model code to be integrated into the execution of the ECU software.
      mask init:
      | ehooks_fcncalltrigger_source_block('mask_init');
      settings: CopyFcn=ehooks_fcncalltrigger_source_block('copy');  DeleteFcn=ehooks_fcncalltrigger_source_block('delete');  UndoDeleteFcn=ehooks_fcncalltrigger_source_block('undo_delete');  ModelCloseFcn=ehooks_fcncalltrigger_source_block('model_close');  PreSaveFcn=ehooks_fcncalltrigger_source_block('pre_save');  PostSaveFcn=ehooks_fcncalltrigger_source_block('post_save');  NameChangeFcn=ehooks_fcncalltrigger_source_block('name_change');  DestroyFcn=ehooks_fcncalltrigger_source_block('destroy', 0); % Second argument just needed to indicate null block. See callback handler.  OpenFcn=ehooks_fcncalltrigger_source_block('open');  CloseFcn=ehooks_fcncalltrigger_source_block('close');  ParentCloseFcn=ehooks_fcncalltrigger_source_block('parent_close');  MoveFcn=ehooks_fcncalltrigger_source_block('move');
      mask Display:
      | image(imread('ehooks_fcncalltrigger_source_small.bmp', 'bmp'), [ 3 1 38 30 ])
      | port_label('Output', 1, 'BypEasyhooks_1ms_Pre_Proc')
  Cpc_flgError : Outport
  Cpc_pChargeFilt : Outport  Port=2
  wires:
  Cpc_calc/1(Cpc_pChargeFilt) -> Cpc_pChargeFilt/1
  Cpc_get/2(Cpc_pMani) -> Cpc_calc/2(Cpc_pMani)
  In1/1 -> Cpc_calc/1(Epm_rpmEngSpd)
  Cpc_pCharge_calc/1(TriggerOut) -> Cpc_calc/Trigger
  Cpc_get/1(Cpc_flgError) -> Cpc_calc/3(Cpc_flgError), Cpc_flgError/1
  Mtc_atMani/1 -> Cpc_get/1(Mtc_atMani)
  Cpc_pCharge_get/1(TriggerOut) -> Cpc_get/Trigger
